simulink model "ejemplo_arduino_pioneer"  (R2016a)
settings: Solver=ode3  StartTime=0.0  StopTime=inf  FixedStep=0.01  RelTol=1e-3
libraries: simulink x2, simulink_extras x1, vrlib x1, sldrtlib x1, aerolibanimutils x1
settings Model: Creator=Usuario  LastModifiedBy=TELEOP
settings DataIOCC: LimitDataPoints=on  SaveFormat=Array
settings DebuggingCC: SolverPrmCheckMsg=warning
settings HardwareCC: ProdBitPerPointer=32  ProdLargestAtomicFloat=None  ProdIntDivRoundTo=Undefined  ProdEndianess=Unspecified  ProdWordSize=32  ProdHWDeviceType=32-bit Generic
settings ModelReferenceCC: PropagateSignalLabelsOutOfModel=off
settings ConfigComp: CovModelRefEnable=Off  CovSFcnEnable=off
settings ConfigurationSet: Description=SimMechanics 2G

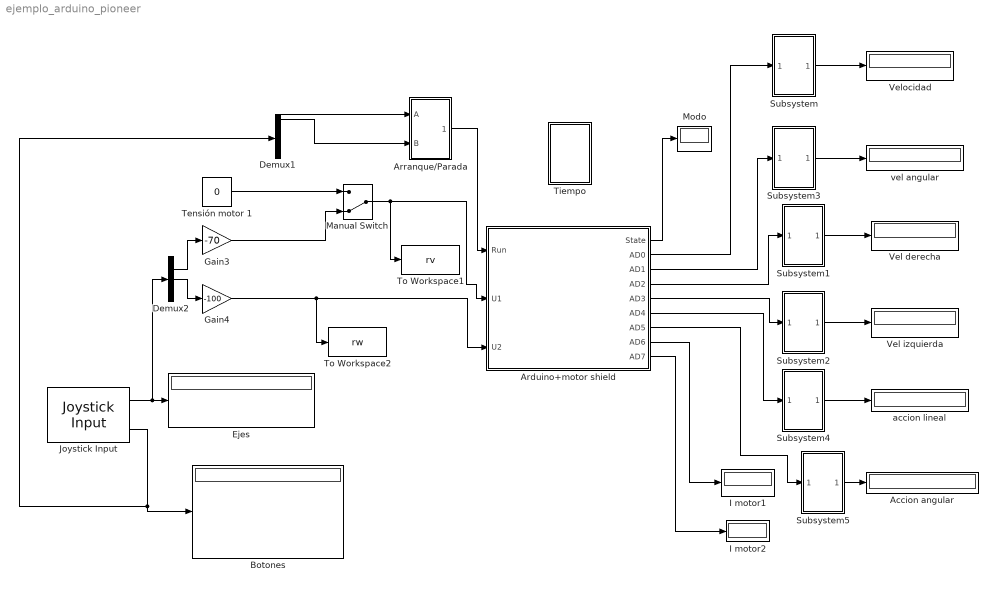
== system ejemplo_arduino_pioneer ==
  Accion angular : Display
  Arduino+motor shield : Subsystem  mask{dev=1}
      mask prompts: dev "Device Number"
      mask Help:
      | HELP DEVICE
      | 
      | - App for using the kit arduino UNO plus Adafruit motor shield 1.2 based on two L293D chips forming 4 H-Bridges. L293D chipset provides 0.6A per bridge (1.2A peak) with thermal shutdown protection, internal kickback protection diodes. Can run motors on 4.5VDC to 25VDC. The shield is compatible with Arduino Mega 1280 & 2560, Diecimila, Duemilanove, and UNO
      | 
      | HELP DRIVERS
      | 
      | Upload the firmware 'Arduino_motor_firmware' in your Arduino UNO kit available from folder '\SAS TOOLS\Software arduino_motor V1.1.0'
      | -------------------------------------------------------------------------------------------------------------------------------------------------------
      | HELP APP
      | 
      | Before running the Simulink model initiate communication with the device through the application 'Arduino_motor.exe' available from folder '\SAS TOOLS\Software arduino_motor V1.1.0'. After executing the program the app icon is available in the taskbar.
      | The app "arduino_motor.exe" is handled from right-click on the icon and selecting the corresponding option:
      | "Play" -> Start the commnunication between the device and the app
      | "Stop" -> Stop the communication
      | "Monitor"->view the state of sensors and communication
      | 
      | -------------------------------------------------------------------------------------------------------------------------------------------------------
      | 
      | HELP BLOCK
      | 
      | Input Ports
      | 
      | Port 'Run': 1 for running and 0 for stopping
      | 
      | Port 'U1': value between [-255;255] which drives the tension applied to the motor 1 of the shield motor Adafruit 1.0
      | Port 'U2': value between [-255;255] which drives the tension applied to the motor 2 of the shield motor Adafruit 1.0
      | Port 'U3': value between [-255;255] which drives the tension applied to the motor 3 of the shield motor Adafruit 1.0
      | Port 'U4': value between [-255;255] which drives the tension applied to the motor 4 of the shield motor Adafruit 1.0
      | 
      | The range [-255;255] is related with the tension range [-V;V], where V is the tension source applied to the motor shield
      | 
      | Output Ports
      | 
      | Port 'State': information about the system. Run=1; Stop=0
      | 
      | Port 'AD0': value between [0;1023] measured in the pin AD0 of the Arduino UNO board
      | Port 'AD1': value between [0;1023] measured in the pin AD1 of the Arduino UNO board
      | Port 'AD2': value between [0;1023] measured in the pin AD2 of the Arduino UNO board
      | Port 'AD3': value between [0;1023] measured in the pin AD3 of the Arduino UNO board
      | 
      | The range [0;1023] is related with the tension range [0;5V] readed on the pins of the Arduino kit A/D conversor
      | -------------------------------------------------------------------------------------------------------------------------------------------------------
      | 
      | HELP SHARE MEMORY (information only for external applications different to "Arduino_motor.exe")
      | 
      | Shared Memory Names:
      | 
      | 'ARDUINO_entrada_'#dev
      | 'ARDUINO_salida_'#dev
      | NOTE: replace #dev with the device number
      mask DialogControl DescGroupVar Prompt: Arduino motor shield
      mask DialogControl DescTextVar Prompt: This block is used to receive and send data via USB port between a UNO Arduino board and the App "Arduino_motor.exe" available on folder '\SAS TOOLS\Software Arduino_motor V1.1.0'. You must upload the firmware "Arduino_motor_firmware" into your Arduino board. More information in Help button.
      mask Display:
      | image('motor_shield.png')
      | color('red')
      | port_label('input',1,'run')
      | port_label('input',2,'U1')
      | port_label('input',3,'U2')
      | port_label('input',4,'U3')
      | port_label('input',5,'U4')
      | color('blue')
      | port_label('output',1,'state')
      | port_label('output',2,'AD0')
      | port_label('output',3,'AD1')
      | port_label('output',4,'AD2')
      | port_label('output',5,'AD3')
  Arranque/Parada : Subsystem
  Botones : Display
  Demux1 : Demux  Outputs=10
  Demux2 : Demux  Outputs=5
  Ejes : Display
  Gain3 : Gain  Gain=-70  OutDataTypeStr=single
  Gain4 : Gain  Gain=-100  OutDataTypeStr=single
  I motor1 : Display
  I motor2 : Display
  Joystick Input : vrlib/Joystick Input  joyid=1  adjustports=on  forcefeed=off
  Manual Switch : ManualSwitch  CurrentSetting=0
  Modo : Display
  Subsystem : Subsystem
  Subsystem1 : Subsystem
  Subsystem2 : Subsystem
  Subsystem3 : Subsystem
  Subsystem4 : Subsystem
  Subsystem5 : Subsystem
  Tensión motor 1 : Constant  Value=0  OutDataTypeStr=single
  Tiempo : Subsystem
  To Workspace1 : ToWorkspace  VariableName=rv  SaveFormat=Timeseries  SampleTime=-1
  To Workspace2 : ToWorkspace  VariableName=rw  SaveFormat=Timeseries  SampleTime=-1
  Vel derecha : Display
  Vel izquierda : Display
  Velocidad : Display
  accion lineal : Display
  vel angular : Display
  wires:
  Gain3/1 -> Manual Switch/2
  Gain4/1 -> Arduino+motor shield/3(U2), To Workspace2/1
  Arduino+motor shield/1(State) -> Modo/1
  Joystick Input/2 -> Demux1/1, Botones/1
  Joystick Input/1 -> Ejes/1, Demux2/1
  Demux2/2 -> Gain3/1
  Demux1/2 -> Arranque/Parada/2(B)
  Arranque/Parada/1(Modo) -> Arduino+motor shield/1(Run)
  Demux2/3 -> Gain4/1
  Tensión motor 1/1 -> Manual Switch/1
  Manual Switch/1 -> To Workspace1/1, Arduino+motor shield/2(U1)
  Arduino+motor shield/8(AD6) -> I motor1/1
  Arduino+motor shield/9(AD7) -> I motor2/1
  Arduino+motor shield/2(AD0) -> Subsystem/1(In1)
  Subsystem/1(Out1) -> Velocidad/1
  Subsystem1/1(Out1) -> Vel derecha/1
  Subsystem2/1(Out1) -> Vel izquierda/1
  Subsystem3/1(Out1) -> vel angular/1
  Arduino+motor shield/6(AD4) -> Subsystem4/1(In1)
  Subsystem4/1(Out1) -> accion lineal/1
  Arduino+motor shield/7(AD5) -> Subsystem5/1(In1)
  Subsystem5/1(Out1) -> Accion angular/1
  Arduino+motor shield/3(AD1) -> Subsystem3/1(In1)
  Arduino+motor shield/4(AD2) -> Subsystem1/1(In1)
  Arduino+motor shield/5(AD3) -> Subsystem2/1(In1)
  Demux1/1 -> Arranque/Parada/1(A)

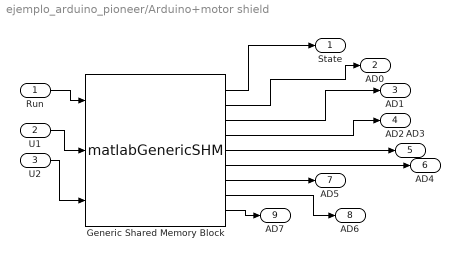
== system ejemplo_arduino_pioneer/Arduino+motor shield ==
  Run : Inport
  U1 : Inport  Port=2
  U2 : Inport  Port=3
  Generic Shared Memory Block : S-Function  FunctionName=matlabGenericSHM  Parameters=nombre,dispositivo,vecE,vecS,tipoE,tipoS  SFunctionDeploymentMode=off  EnableBusSupport=off  mask(Generic Share Memory block V2.0){nombre='ARDUINO', dispositivo=dev, vecE=[1 1 1], vecS=[1 1 1 1 1 1 1 1 1], tipoE=['f' 'f' 'f'], tipoS=['f' 'f' 'f' 'f' 'f' 'f' 'f' 'f' 'f' ]}
      mask prompts: nombre "Share Memory base name"; dispositivo "Device Number"; vecE "Sizes input vector"; vecS "Sizes output vector"; tipoE "Data Types Inputs"; tipoS "Data Types Outputs"
      mask help:
      | This block allows Simulink communication with external processes through shared memory. It works on Unix and Windows.
      | More information in Help.
      mask Help:
      | Share Memory base name (nombre): It's the base string of share memory ej 'robot'
      | Device Number (dispositivo): integer that identifies the device between multiple in use
      | Two shared memorys are created with names:
      | "%name_entrada_%dispositivo" for the device input (writing)
      | "%name_salida_%dispositivo" for the device output (reading)
      | Sizes input vector (vecE)  : array that specify the number of inputs (array dimension) and the inputs size (array values)
      | Sizes output vector  (vecS): array that specify the number of outputs (array dimension) and the outputs size (array values)
      | Data types input(tipoE): char array that specify each input types
      | Data types output (tipoS): char array that specify each output types
      | Allowed types are:
      | ('f'=float, 'd'=double, 'i'=int32, 'c'=char, 'C'= unsigned char, 'I'=unsigned int)
      | Example.
      | Suppose the following parameters:
      | nombre='exampleMemory'
      | dispositivo=10
      | vecE=[3 2 1]
      | vecS=[6 5 7 8]
      | tipoE=['f' 'I' 'c']
      | tipoS=['C' 'i' 'd' 'd']
      | 
      | Two Share Memories are created with names:
      | "exampleMemory_entrada_10" (block input)
      | "exampleMemory_salida_10"  (block output)
      | 3 inputs are created:
      |  1° Dimension 3, type "unsigned char"
      |  2° Dimension 2, type "int"
      |  3° Dimension 1, type "char"
      | 4 outputs are created:
      |  1° Dimension 6, type "float"
      |  2° Dimension 5, type "unsigned int"
      |  3° Dimension 7, type "double"
      |  3° Dimension 8, type "double"
      mask Display: image('shmem.jpg')
  State : Outport
  AD0 : Outport  Port=2
  AD1 : Outport  Port=3
  AD2 : Outport  Port=4
  AD3 : Outport  Port=5
  AD4 : Outport  Port=6
  AD5 : Outport  Port=7
  AD6 : Outport  Port=8
  AD7 : Outport  Port=9
  wires:
  Generic Shared Memory Block/5 -> AD3/1
  Generic Shared Memory Block/4 -> AD2/1
  Generic Shared Memory Block/3 -> AD1/1
  Generic Shared Memory Block/2 -> AD0/1
  Generic Shared Memory Block/1 -> State/1
  U2/1 -> Generic Shared Memory Block/3
  U1/1 -> Generic Shared Memory Block/2
  Run/1 -> Generic Shared Memory Block/1
  Generic Shared Memory Block/9 -> AD7/1
  Generic Shared Memory Block/8 -> AD6/1
  Generic Shared Memory Block/7 -> AD5/1
  Generic Shared Memory Block/6 -> AD4/1

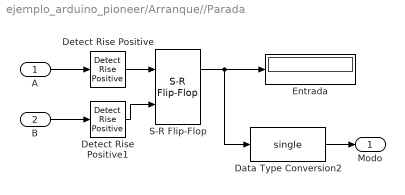
== system ejemplo_arduino_pioneer/Arranque//Parada ==
  A : Inport
  B : Inport  Port=2
  Data Type Conversion2 : DataTypeConversion  OutDataTypeStr=single
  Detect Rise Positive : simulink/Logic and Bit Operations/Detect Rise Positive  vinit=0  InputProcessing=Inherited  OutDataTypeStr=boolean
  Detect Rise Positive1 : simulink/Logic and Bit Operations/Detect Rise Positive  vinit=0  InputProcessing=Inherited  OutDataTypeStr=boolean
  Entrada : Display
  S-R Flip-Flop : simulink_extras/Flip Flops/S-R Flip-Flop  initial_condition=0
  Modo : Outport
  wires:
  B/1 -> Detect Rise Positive1/1
  S-R Flip-Flop/1 -> Entrada/1, Data Type Conversion2/1
  Detect Rise Positive/1 -> S-R Flip-Flop/1
  Data Type Conversion2/1 -> Modo/1
  Detect Rise Positive1/1 -> S-R Flip-Flop/2
  A/1 -> Detect Rise Positive/1

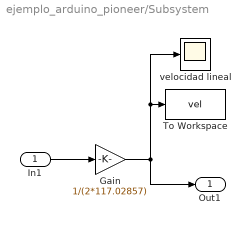
== system ejemplo_arduino_pioneer/Subsystem ==
  In1 : Inport
  Gain : Gain  Gain=1/(2*117.02857)
  To Workspace : ToWorkspace  VariableName=vel  SaveFormat=Timeseries  SampleTime=-1
  velocidad lineal : Scope
  Out1 : Outport
  wires:
  Gain/1 -> Out1/1, To Workspace/1, velocidad lineal/1
  In1/1 -> Gain/1

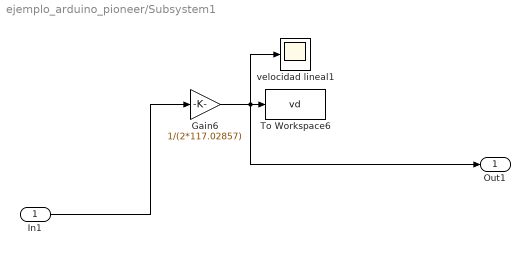
== system ejemplo_arduino_pioneer/Subsystem1 ==
  In1 : Inport
  Gain6 : Gain  Gain=1/(2*117.02857)
  To Workspace6 : ToWorkspace  VariableName=vd  SaveFormat=Timeseries  SampleTime=-1
  velocidad lineal1 : Scope
  Out1 : Outport
  wires:
  In1/1 -> Gain6/1
  Gain6/1 -> Out1/1, velocidad lineal1/1, To Workspace6/1

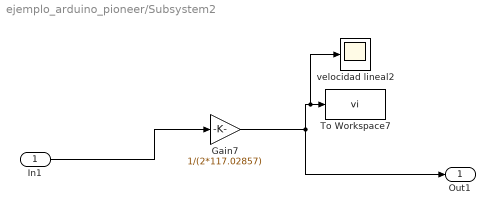
== system ejemplo_arduino_pioneer/Subsystem2 ==
  In1 : Inport
  Gain7 : Gain  Gain=1/(2*117.02857)
  To Workspace7 : ToWorkspace  VariableName=vi  SaveFormat=Timeseries  SampleTime=-1
  velocidad lineal2 : Scope
  Out1 : Outport
  wires:
  In1/1 -> Gain7/1
  Gain7/1 -> Out1/1, To Workspace7/1, velocidad lineal2/1

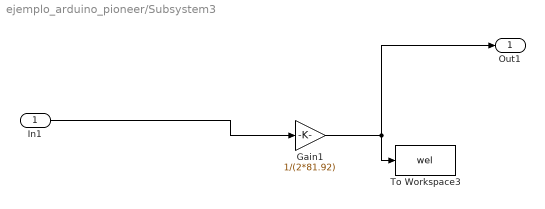
== system ejemplo_arduino_pioneer/Subsystem3 ==
  In1 : Inport
  Gain1 : Gain  Gain=1/(2*81.92)  ParamDataTypeStr=double
  To Workspace3 : ToWorkspace  VariableName=wel  SaveFormat=Timeseries  SampleTime=-1
  Out1 : Outport
  wires:
  Gain1/1 -> Out1/1, To Workspace3/1
  In1/1 -> Gain1/1

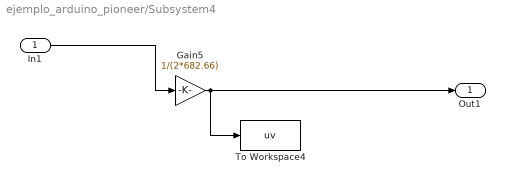
== system ejemplo_arduino_pioneer/Subsystem4 ==
  In1 : Inport
  Gain5 : Gain  Gain=1/(2*682.66)
  To Workspace4 : ToWorkspace  VariableName=uv  SaveFormat=Timeseries  SampleTime=-1
  Out1 : Outport
  wires:
  Gain5/1 -> Out1/1, To Workspace4/1
  In1/1 -> Gain5/1

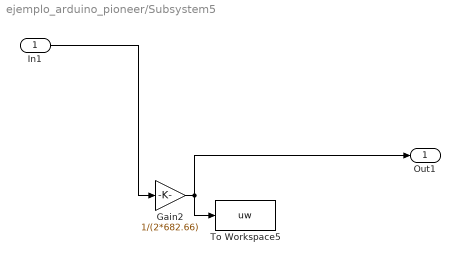
== system ejemplo_arduino_pioneer/Subsystem5 ==
  In1 : Inport
  Gain2 : Gain  Gain=1/(2*682.66)
  To Workspace5 : ToWorkspace  VariableName=uw  SaveFormat=Timeseries  SampleTime=-1
  Out1 : Outport
  wires:
  Gain2/1 -> Out1/1, To Workspace5/1
  In1/1 -> Gain2/1

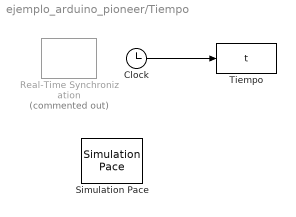
== system ejemplo_arduino_pioneer/Tiempo ==
  Clock : Clock
  Real-Time Synchronization : sldrtlib/Real-Time Synchronization  Commented=on  SampleTime=0.01  MaxMissedTicks=inf  ShowMissedTicks=off  YieldWhenWaiting=off
  Simulation Pace : aerolibanimutils/Simulation Pace  SimulationPace=1  SleepMode=MATLAB Thread  OutputPaceError=off  SampleTime=0.1
  Tiempo : ToWorkspace  VariableName=t  SampleTime=-1
  wires:
  Clock/1 -> Tiempo/1
